simulink model "SalirClaseWaypointsMF"  (R2022b)
settings: Solver=VariableStepAuto  StartTime=0.0  StopTime=10.0  RelTol=1e-3
libraries: slpidlib x1, robotalgslib x1
settings Model: Creator=Usuario_UMA  LastModifiedBy=Usuario_UMA

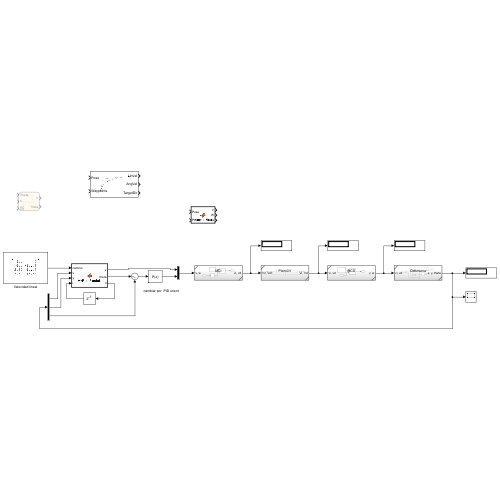
[thumbnail: Simulink's stored preview of the top-level diagram]
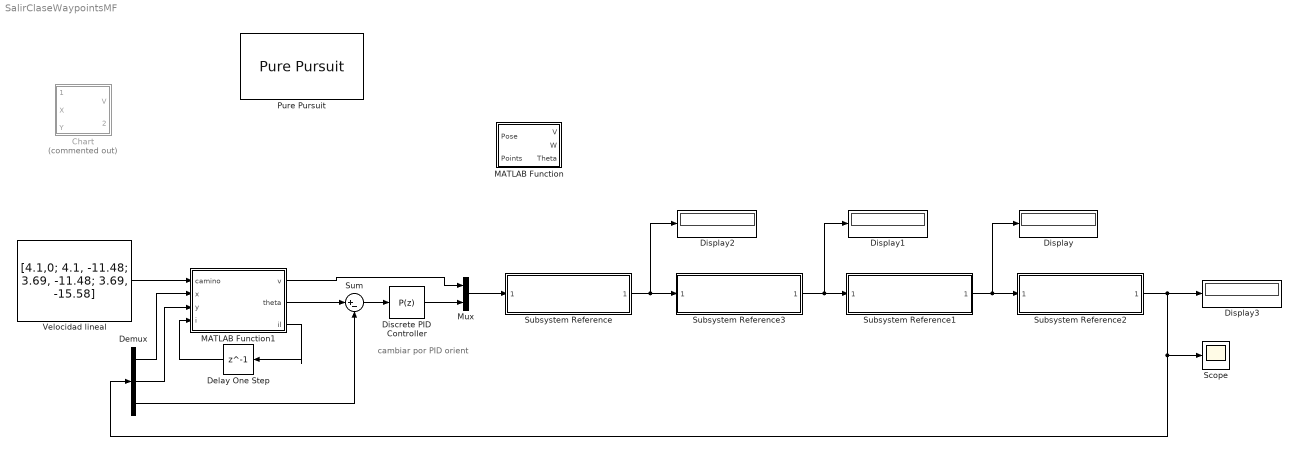
== system SalirClaseWaypointsMF ==
  note: cambiar por PID orient
  Chart : Stateflow chart  Commented=on  TreatAsAtomicUnit=on
  Delay One Step : Delay  DelayLength=1
  Demux : Demux  Outputs=3
  Discrete PID Controller : slpidlib/PID Controller  Controller=P  Form=Parallel  TimeDomain=Discrete-time  UseExternalTs=off  SampleTime=-1  IntegratorMethod=Forward Euler  FilterMethod=Forward Euler  ControllerParametersSource=internal  P=1  I=1  UseKiTs=off  D=0  N=100  UseFilter=on  TunerSelectOption=Transfer Function Based (PID Tuner App)  InitialConditionSource=internal  InitialConditionForIntegrator=0  InitialConditionForFilter=0  DifferentiatorICPrevScaledInput=0  ExternalReset=none  TrackingMode=off  Kt=1  LimitOutput=off  SatLimitsSource=internal  UpperSaturationLimit=inf  LowerSaturationLimit=-inf  LinearizeAsGain=off  AntiWindupMode=none  Kb=1  LimitIntegrator=off  UpperIntegratorSaturationLimit=inf  LowerIntegratorSaturationLimit=-inf  POutMin=[]  POutMax=[]  IOutMin=[]  IOutMax=[]  DOutMin=[]  DOutMax=[]  NOutMin=[]  NOutMax=[]  SumOutMin=[]  SumOutMax=[]  SaturationOutMin=[]  SaturationOutMax=[]  PParamMin=[]  PParamMax=[]  IParamMin=[]  IParamMax=[]  DParamMin=[]  DParamMax=[]  NParamMin=[]  NParamMax=[]  KbParamMin=[]  KbParamMax=[]  KtParamMin=[]  KtParamMax=[]  KbOutMin=[]  KbOutMax=[]  KtOutMin=[]  KtOutMax=[]  IntegratorOutMin=[]  IntegratorOutMax=[]  FilterOutMin=[]  FilterOutMax=[]  SumI1OutMin=[]  SumI1OutMax=[]  SumI2OutMin=[]  SumI2OutMax=[]  SumI3OutMin=[]  SumI3OutMax=[]  SumI4OutMin=[]  SumI4OutMax=[]  SumDOutMin=[]  SumDOutMax=[]  DifferentiatorOutMin=[]  DifferentiatorOutMax=[]  FilterDiffOutCoefMin=[]  FilterDiffOutCoefMax=[]  ReciprocalOutMin=[]  ReciprocalOutMax=[]  SumDenOutMin=[]  SumDenOutMax=[]  SumNumOutMin=[]  SumNumOutMax=[]  DivideOutMin=[]  DivideOutMax=[]  UdiffTsProdOutMin=[]  UdiffTsProdOutMax=[]  NTsProdOutMin=[]  NTsProdOutMax=[]  UintegralTsProdOutMin=[]  UintegralTsProdOutMax=[]  UngainTsProdOutMin=[]  UngainTsProdOutMax=[]  ClampingZeroOutDataTypeStr=Inherit: Inherit via back propagation  ClampingZeroOutMin=[]  ClampingZeroOutMax=[]  FilterDenConstantOutDataTypeStr=Inherit: Inherit via back propagation  FilterDenConstantOutMin=[]  FilterDenConstantOutMax=[]  PCopyOutDataTypeStr=Inherit: Inherit via back propagation  PCopyOutMin=[]  PCopyOutMax=[]  NCopyOutDataTypeStr=Inherit: Inherit via back propagation  NCopyOutMin=[]  NCopyOutMax=[]  IntegratorContinuousStateAttributes=''  IntegratorStateMustResolveToSignalObject=off  IntegratorRTWStateStorageClass=Auto  FilterContinuousStateAttributes=''  FilterStateMustResolveToSignalObject=off  FilterRTWStateStorageClass=Auto  ParallelPVariant=InternalParameters  IdealPVariant=Disabled  IVariant=Disabled  DVariant=Disabled  IntegratorVariant=Disabled  SatVariant=Disabled  AWVariant=Disabled  PCopyVariant=Disabled  TRVariant=Disabled  FdbkBlocksVariant=Forward  IdealPFdbkVariant=Disabled  SatFdbkVariant=Disabled  DerivativeFilterVariant=Disabled  NVariant=Disabled  NCopyVariant=Disabled_SignalSpec  FilterICVariant=Disabled  IntegratorICVariant=Disabled  ExternalResetVariant=Disabled  TRSumVariant=Passthrough  SumFdbkVariant=Disabled  SumVariant=Passthrough_P  TsampFilterVariant=InternalTs  TsampNgainVariant=Passthrough  TsampIntegralVariant=Disabled_SignalSpec  ExternalSaturationOutDataTypeStr=Inherit: Same as second input
      settings: LibrarySourceBlock=simulink/Discrete/Discrete PID Controller
  Display{,1..3} (4 alike) : Display
  MATLAB Function : MATLAB Function  TreatAsAtomicUnit=on
  MATLAB Function1 : MATLAB Function  TreatAsAtomicUnit=on
  Mux : Mux  Inputs=2
  Pure Pursuit : robotalgslib/Pure Pursuit  DesiredLinearVelocity=0.1  MaxAngularVelocity=1.0  LookaheadDistance=1.0  TargetDirPort=on  SimulateUsing=Code generation
      settings: LibrarySourceBlock=navlib/Control Algorithms/Pure Pursuit
  Scope : Scope
  Subsystem Reference : Subsystem  ReferencedSubsystem=MCI
  Subsystem Reference1 : Subsystem  ReferencedSubsystem=MCD
  Subsystem Reference2 : Subsystem  ReferencedSubsystem=Odometria
  Subsystem Reference3 : Subsystem  ReferencedSubsystem=PieroCV
  Sum : Sum  Inputs=|+-
  Velocidad lineal : Constant  Value=[4.1,0; 4.1, -11.48; 3.69, -11.48; 3.69, -15.58]
  wires:
  Discrete PID Controller/1 -> Mux/2
  Subsystem Reference3/1 -> Display1/1, Subsystem Reference1/1
  Subsystem Reference2/1 -> Scope/1, Demux/1, Display3/1
  Sum/1 -> Discrete PID Controller/1
  Demux/3 -> Sum/2
  Subsystem Reference1/1 -> Display/1, Subsystem Reference2/1
  Mux/1 -> Subsystem Reference/1
  Subsystem Reference/1 -> Display2/1, Subsystem Reference3/1
  MATLAB Function1/3(il) -> Delay One Step/1
  Delay One Step/1 -> MATLAB Function1/4(i)
  MATLAB Function1/2(theta) -> Sum/1
  MATLAB Function1/1(v) -> Mux/1
  Velocidad lineal/1 -> MATLAB Function1/1(camino)
  Demux/1 -> MATLAB Function1/2(x)
  Demux/2 -> MATLAB Function1/3(y)

== matlab function SalirClaseWaypointsMF/MATLAB Function1 ==
  data: camino input; v output; x input; y input; i input; theta output; il output
function [v,theta,il] = HyPurePerduit(camino,x,y,i)
L = 0.15; %Distancia de persecution 
v = 0.205; 
theta = 0; 
i = i+1;
if length(camino) >=i %Mientras haya camino 
    %Calculamos distancia al objetivo 
    distancia = sqrt((camino(i,1)-x)^2 + (camino(i,2)-y)^2);
    while(distancia<0)&&(length(camino)>i)% ya hemos 
        i = i+1; %Actualizar objetivo 
        distancia = sqrt((camino(i,1)-x)^2 + (camino(i,2)-y)^2); 
        v = 0.205; 
    end 
    %Calculo de la orientation al punto i-esimo 
    theta = atan2((camino(i,2)-y),(camino(i,1)-x)); 
else %si ha Ilegado al objetivo final se para
    theta = 0;
    v = 0; 
end 

if i<(length(camino))
    il = i - 1; 
else 
    il = 1; 
end 
end

== matlab function SalirClaseWaypointsMF/MATLAB Function ==
  data: Pose input; V output; Points input; W output; Theta output
function [V, W, Theta] = PurePursuit(Pose, Points)
x = Points(:,1)';
y = Points(:,2)';

robot_x = Pose(1);
robot_y = Pose(2);
robot_theta = Pose(3);

n = length(x);

lookahead = 0.2;    %umbral de cambio al siguiente punto
linear_vel = 0.205; w_max = 1.5;

persistent index;
if isempty(index)
    index = 1;
end

if (index < n)
    target_x = x(index);
    target_y = y(index);
    
    % Distancia y ángulo al punto objetivo
    distance = sqrt((target_x - robot_x)^2 + (target_y - robot_y)^2);
    angle = atan2(target_y - robot_y, target_x - robot_x) - robot_theta;
    
    if distance < lookahead     % Cambiar por un while
        index = index +1;
    end

    Theta = angle;
    V = linear_vel;

    if (lookahead < 1.0)
        R = ((lookahead+0.1)/(2*sin(angle)));
    else
        R = (lookahead/(2*sin(angle)));
    end

    W = 0.25 / R;

    if (W > w_max)
        W = w_max;
    end
else
    W = 0;  V = 0;

end

end

== stateflow chart SalirClaseWaypointsMF/Chart ==
  state Paro
    V=0;
    Theta=0;
  state Tramo10A
    entry:
    V=0.205;
    Theta=0;
  state GiroDer1
    entry:
    V=0.05;
    Theta=-pi/2;
  state Tramo28A
    entry:
    V=0.205;
    Theta=-pi/2;
  state GiroDer3
    entry:
    V=0.05;
    Theta=-pi/2;
  state Tramo1A
    entry:
    V=0.205;
    Theta=0;
  state GiroDer2
    entry:
    V=0.05;
    Theta=-pi;
  state Tramo10A2
    entry:
    V=0.205;
    Theta=-pi/2;
  state FIN
    entry:
    V=0;
    Theta=-pi/2;
  (default) -> Paro
  Paro -> Tramo10A : after(2,sec)
  Tramo10A -> GiroDer1 : [X>=4.1]
  GiroDer1 -> Tramo28A : [iTheta<=(-pi/2)]
  Tramo28A -> GiroDer2 : [Y<=-11.48]
  Tramo1A -> GiroDer3 : [X<=3.69]
  GiroDer2 -> Tramo1A : [iTheta<=-pi]
  GiroDer3 -> Tramo10A2 : [iTheta>=(-pi/2)]
  Tramo10A2 -> FIN : [Y<=-15.58]
  data: iTheta input; X input; Y input; V output; Theta output
